simulink model "x5_Click"  (R2024b)
settings: Solver=VariableStepAuto  StartTime=0.0  StopTime=inf  RelTol=1e-3  EnableMultiTasking=on
libraries: simulink x6
(part 3 of 3)

== matlab function x5_Click/Robot_Direct_Kinematics1 ==
  data: q1 input; R06 output; q2 input; q3 input; q4 input; q5 input; q6 input; P6 output; J output
function [R06,P6,J] = Robot_Direct_Kinematics(q1,q2,q3,q4,q5,q6)
%#codegen

%    This function was generated by the Symbolic Math Toolbox version 24.2.
%    21-May-2025 19:19:44

% q1 = complex(q1);  % if required to enforce complex operations
% q2 = complex(q2);  % if required to enforce complex operations
% q3 = complex(q3);  % if required to enforce complex operations
% q4 = complex(q4);  % if required to enforce complex operations
% q5 = complex(q5);  % if required to enforce complex operations
% q6 = complex(q6);  % if required to enforce complex operations
et1 = cos(q5).*sin(q1).*sin(q3).*sqrt(sqrt(2.0)+2.0).*(-1.0./2.0)-(cos(q1).*cos(q2).*sin(q4).*sin(q6).*sqrt(-sqrt(2.0)+2.0))./2.0-(cos(q3).*cos(q4).*sin(q1).*sin(q6).*sqrt(-sqrt(2.0)+2.0))./2.0-(cos(q6).*sin(q1).*sin(q3).*sin(q5).*sqrt(-sqrt(2.0)+2.0))./2.0-(cos(q1).*cos(q3).*cos(q5).*sin(q2).*sqrt(sqrt(2.0)+2.0))./2.0-(cos(q1).*cos(q2).*cos(q4).*sin(q5).*sqrt(sqrt(2.0)+2.0))./2.0+(cos(q3).*sin(q1).*sin(q4).*sin(q5).*sqrt(sqrt(2.0)+2.0))./2.0;
et2 = (cos(q1).*cos(q2).*cos(q4).*cos(q5).*cos(q6).*sqrt(-sqrt(2.0)+2.0))./2.0-(cos(q1).*cos(q3).*cos(q6).*sin(q2).*sin(q5).*sqrt(-sqrt(2.0)+2.0))./2.0-(cos(q3).*cos(q5).*cos(q6).*sin(q1).*sin(q4).*sqrt(-sqrt(2.0)+2.0))./2.0+(cos(q1).*cos(q4).*sin(q2).*sin(q3).*sin(q6).*sqrt(-sqrt(2.0)+2.0))./2.0-(cos(q1).*sin(q2).*sin(q3).*sin(q4).*sin(q5).*sqrt(sqrt(2.0)+2.0))./2.0+(cos(q1).*cos(q5).*cos(q6).*sin(q2).*sin(q3).*sin(q4).*sqrt(-sqrt(2.0)+2.0))./2.0;
et3 = cos(q1).*cos(q5).*sin(q3).*sqrt(sqrt(2.0)+2.0).*(-1.0./2.0)-(cos(q1).*cos(q3).*cos(q4).*sin(q6).*sqrt(-sqrt(2.0)+2.0))./2.0-(cos(q1).*cos(q6).*sin(q3).*sin(q5).*sqrt(-sqrt(2.0)+2.0))./2.0+(cos(q2).*sin(q1).*sin(q4).*sin(q6).*sqrt(-sqrt(2.0)+2.0))./2.0+(cos(q3).*cos(q5).*sin(q1).*sin(q2).*sqrt(sqrt(2.0)+2.0))./2.0+(cos(q2).*cos(q4).*sin(q1).*sin(q5).*sqrt(sqrt(2.0)+2.0))./2.0+(cos(q1).*cos(q3).*sin(q4).*sin(q5).*sqrt(sqrt(2.0)+2.0))./2.0-(cos(q2).*cos(q4).*cos(q5).*cos(q6).*sin(q1).*sqrt(-sqrt(2.0)+2.0))./2.0;
et4 = cos(q1).*cos(q3).*cos(q5).*cos(q6).*sin(q4).*sqrt(-sqrt(2.0)+2.0).*(-1.0./2.0)+(cos(q3).*cos(q6).*sin(q1).*sin(q2).*sin(q5).*sqrt(-sqrt(2.0)+2.0))./2.0-(cos(q4).*sin(q1).*sin(q2).*sin(q3).*sin(q6).*sqrt(-sqrt(2.0)+2.0))./2.0+(sin(q1).*sin(q2).*sin(q3).*sin(q4).*sin(q5).*sqrt(sqrt(2.0)+2.0))./2.0-(cos(q5).*cos(q6).*sin(q1).*sin(q2).*sin(q3).*sin(q4).*sqrt(-sqrt(2.0)+2.0))./2.0;
et5 = cos(q5).*sin(q1).*sin(q3).*sqrt(-sqrt(2.0)+2.0).*(-1.0./2.0)-(cos(q1).*cos(q3).*cos(q5).*sin(q2).*sqrt(-sqrt(2.0)+2.0))./2.0-(cos(q1).*cos(q2).*cos(q4).*sin(q5).*sqrt(-sqrt(2.0)+2.0))./2.0+(cos(q3).*sin(q1).*sin(q4).*sin(q5).*sqrt(-sqrt(2.0)+2.0))./2.0+(cos(q1).*cos(q2).*sin(q4).*sin(q6).*sqrt(sqrt(2.0)+2.0))./2.0+(cos(q3).*cos(q4).*sin(q1).*sin(q6).*sqrt(sqrt(2.0)+2.0))./2.0+(cos(q6).*sin(q1).*sin(q3).*sin(q5).*sqrt(sqrt(2.0)+2.0))./2.0;
et6 = cos(q1).*sin(q2).*sin(q3).*sin(q4).*sin(q5).*sqrt(-sqrt(2.0)+2.0).*(-1.0./2.0)-(cos(q1).*cos(q2).*cos(q4).*cos(q5).*cos(q6).*sqrt(sqrt(2.0)+2.0))./2.0+(cos(q1).*cos(q3).*cos(q6).*sin(q2).*sin(q5).*sqrt(sqrt(2.0)+2.0))./2.0+(cos(q3).*cos(q5).*cos(q6).*sin(q1).*sin(q4).*sqrt(sqrt(2.0)+2.0))./2.0-(cos(q1).*cos(q4).*sin(q2).*sin(q3).*sin(q6).*sqrt(sqrt(2.0)+2.0))./2.0-(cos(q1).*cos(q5).*cos(q6).*sin(q2).*sin(q3).*sin(q4).*sqrt(sqrt(2.0)+2.0))./2.0;
et7 = cos(q1).*cos(q5).*sin(q3).*sqrt(-sqrt(2.0)+2.0).*(-1.0./2.0)+(cos(q3).*cos(q5).*sin(q1).*sin(q2).*sqrt(-sqrt(2.0)+2.0))./2.0+(cos(q2).*cos(q4).*sin(q1).*sin(q5).*sqrt(-sqrt(2.0)+2.0))./2.0+(cos(q1).*cos(q3).*sin(q4).*sin(q5).*sqrt(-sqrt(2.0)+2.0))./2.0+(cos(q1).*cos(q3).*cos(q4).*sin(q6).*sqrt(sqrt(2.0)+2.0))./2.0+(cos(q1).*cos(q6).*sin(q3).*sin(q5).*sqrt(sqrt(2.0)+2.0))./2.0-(cos(q2).*sin(q1).*sin(q4).*sin(q6).*sqrt(sqrt(2.0)+2.0))./2.0;
et8 = (sin(q1).*sin(q2).*sin(q3).*sin(q4).*sin(q5).*sqrt(-sqrt(2.0)+2.0))./2.0+(cos(q2).*cos(q4).*cos(q5).*cos(q6).*sin(q1).*sqrt(sqrt(2.0)+2.0))./2.0+(cos(q1).*cos(q3).*cos(q5).*cos(q6).*sin(q4).*sqrt(sqrt(2.0)+2.0))./2.0-(cos(q3).*cos(q6).*sin(q1).*sin(q2).*sin(q5).*sqrt(sqrt(2.0)+2.0))./2.0+(cos(q4).*sin(q1).*sin(q2).*sin(q3).*sin(q6).*sqrt(sqrt(2.0)+2.0))./2.0+(cos(q5).*cos(q6).*sin(q1).*sin(q2).*sin(q3).*sin(q4).*sqrt(sqrt(2.0)+2.0))./2.0;
mt1 = [cos(q1).*cos(q3).*cos(q4).*cos(q6)-cos(q2).*cos(q6).*sin(q1).*sin(q4)-cos(q1).*sin(q3).*sin(q5).*sin(q6)-cos(q2).*cos(q4).*cos(q5).*sin(q1).*sin(q6)-cos(q1).*cos(q3).*cos(q5).*sin(q4).*sin(q6)+cos(q4).*cos(q6).*sin(q1).*sin(q2).*sin(q3)+cos(q3).*sin(q1).*sin(q2).*sin(q5).*sin(q6)-cos(q5).*sin(q1).*sin(q2).*sin(q3).*sin(q4).*sin(q6),cos(q1).*cos(q2).*cos(q6).*sin(q4)+cos(q3).*cos(q4).*cos(q6).*sin(q1)-sin(q1).*sin(q3).*sin(q5).*sin(q6)+cos(q1).*cos(q2).*cos(q4).*cos(q5).*sin(q6)-cos(q1).*cos(q4).*cos(q6).*sin(q2).*sin(q3)-cos(q1).*cos(q3).*sin(q2).*sin(q5).*sin(q6)-cos(q3).*cos(q5).*sin(q1).*sin(q4).*sin(q6)+cos(q1).*cos(q5).*sin(q2).*sin(q3).*sin(q4).*sin(q6)];
mt2 = [cos(q6).*sin(q2).*sin(q4)+cos(q2).*cos(q4).*cos(q6).*sin(q3)+cos(q2).*cos(q3).*sin(q5).*sin(q6)+cos(q4).*cos(q5).*sin(q2).*sin(q6)-cos(q2).*cos(q5).*sin(q3).*sin(q4).*sin(q6),et3+et4,et1+et2];
mt3 = [cos(q4).*sin(q2).*sin(q5).*sqrt(sqrt(2.0)+2.0).*(-1.0./2.0)-(sin(q2).*sin(q4).*sin(q6).*sqrt(-sqrt(2.0)+2.0))./2.0+(cos(q2).*cos(q3).*cos(q5).*sqrt(sqrt(2.0)+2.0))./2.0+(cos(q2).*cos(q3).*cos(q6).*sin(q5).*sqrt(-sqrt(2.0)+2.0))./2.0+(cos(q4).*cos(q5).*cos(q6).*sin(q2).*sqrt(-sqrt(2.0)+2.0))./2.0-(cos(q2).*cos(q4).*sin(q3).*sin(q6).*sqrt(-sqrt(2.0)+2.0))./2.0+(cos(q2).*sin(q3).*sin(q4).*sin(q5).*sqrt(sqrt(2.0)+2.0))./2.0-(cos(q2).*cos(q5).*cos(q6).*sin(q3).*sin(q4).*sqrt(-sqrt(2.0)+2.0))./2.0];
mt4 = [et7+et8,et5+et6,(sin(q2).*sin(q4).*sin(q6).*sqrt(sqrt(2.0)+2.0))./2.0+(cos(q2).*cos(q3).*cos(q5).*sqrt(-sqrt(2.0)+2.0))./2.0-(cos(q4).*sin(q2).*sin(q5).*sqrt(-sqrt(2.0)+2.0))./2.0+(cos(q2).*sin(q3).*sin(q4).*sin(q5).*sqrt(-sqrt(2.0)+2.0))./2.0-(cos(q2).*cos(q3).*cos(q6).*sin(q5).*sqrt(sqrt(2.0)+2.0))./2.0-(cos(q4).*cos(q5).*cos(q6).*sin(q2).*sqrt(sqrt(2.0)+2.0))./2.0+(cos(q2).*cos(q4).*sin(q3).*sin(q6).*sqrt(sqrt(2.0)+2.0))./2.0+(cos(q2).*cos(q5).*cos(q6).*sin(q3).*sin(q4).*sqrt(sqrt(2.0)+2.0))./2.0];
R06 = reshape([mt1,mt2,mt3,mt4],3,3);
if nargout > 1
    et9 = sin(q2).*(-2.0./5.0)+(cos(q4).*sin(q2))./1.0e+1+(sin(q2).*sin(q4))./2.0+(cos(q2).*cos(q3).*cos(q5))./1.0e+1+(cos(q2).*cos(q4).*sin(q3))./2.0-(cos(q2).*sin(q3).*sin(q4))./1.0e+1-(cos(q4).*sin(q2).*sin(q5))./1.0e+1+sin(q2).*sin(q4).*sin(q6).*sqrt(sqrt(2.0)+2.0).*(3.0./4.0e+1)+cos(q2).*cos(q3).*cos(q5).*sqrt(-sqrt(2.0)+2.0).*(3.0./4.0e+1)-cos(q4).*sin(q2).*sin(q5).*sqrt(-sqrt(2.0)+2.0).*(3.0./4.0e+1)+(cos(q2).*sin(q3).*sin(q4).*sin(q5))./1.0e+1+cos(q2).*sin(q3).*sin(q4).*sin(q5).*sqrt(-sqrt(2.0)+2.0).*(3.0./4.0e+1);
    et10 = cos(q2).*cos(q3).*cos(q6).*sin(q5).*sqrt(sqrt(2.0)+2.0).*(-3.0./4.0e+1)-cos(q4).*cos(q5).*cos(q6).*sin(q2).*sqrt(sqrt(2.0)+2.0).*(3.0./4.0e+1)+cos(q2).*cos(q4).*sin(q3).*sin(q6).*sqrt(sqrt(2.0)+2.0).*(3.0./4.0e+1)+cos(q2).*cos(q5).*cos(q6).*sin(q3).*sin(q4).*sqrt(sqrt(2.0)+2.0).*(3.0./4.0e+1);
    et11 = cos(q1).*cos(q2).*(-2.0./5.0)+(cos(q1).*cos(q2).*cos(q4))./1.0e+1+(cos(q1).*cos(q2).*sin(q4))./2.0+(cos(q3).*cos(q4).*sin(q1))./2.0-(cos(q3).*sin(q1).*sin(q4))./1.0e+1-(cos(q5).*sin(q1).*sin(q3))./1.0e+1-cos(q5).*sin(q1).*sin(q3).*sqrt(-sqrt(2.0)+2.0).*(3.0./4.0e+1)-(cos(q1).*cos(q3).*cos(q5).*sin(q2))./1.0e+1-(cos(q1).*cos(q2).*cos(q4).*sin(q5))./1.0e+1-(cos(q1).*cos(q4).*sin(q2).*sin(q3))./2.0+(cos(q1).*sin(q2).*sin(q3).*sin(q4))./1.0e+1+(cos(q3).*sin(q1).*sin(q4).*sin(q5))./1.0e+1-cos(q1).*cos(q3).*cos(q5).*sin(q2).*sqrt(-sqrt(2.0)+2.0).*(3.0./4.0e+1);
    et12 = cos(q1).*cos(q2).*cos(q4).*sin(q5).*sqrt(-sqrt(2.0)+2.0).*(-3.0./4.0e+1)+cos(q3).*sin(q1).*sin(q4).*sin(q5).*sqrt(-sqrt(2.0)+2.0).*(3.0./4.0e+1)-(cos(q1).*sin(q2).*sin(q3).*sin(q4).*sin(q5))./1.0e+1+cos(q1).*cos(q2).*sin(q4).*sin(q6).*sqrt(sqrt(2.0)+2.0).*(3.0./4.0e+1)+cos(q3).*cos(q4).*sin(q1).*sin(q6).*sqrt(sqrt(2.0)+2.0).*(3.0./4.0e+1)+cos(q6).*sin(q1).*sin(q3).*sin(q5).*sqrt(sqrt(2.0)+2.0).*(3.0./4.0e+1)-cos(q1).*sin(q2).*sin(q3).*sin(q4).*sin(q5).*sqrt(-sqrt(2.0)+2.0).*(3.0./4.0e+1)-cos(q1).*cos(q2).*cos(q4).*cos(q5).*cos(q6).*sqrt(sqrt(2.0)+2.0).*(3.0./4.0e+1);
    et13 = cos(q1).*cos(q3).*cos(q6).*sin(q2).*sin(q5).*sqrt(sqrt(2.0)+2.0).*(3.0./4.0e+1)+cos(q3).*cos(q5).*cos(q6).*sin(q1).*sin(q4).*sqrt(sqrt(2.0)+2.0).*(3.0./4.0e+1)-cos(q1).*cos(q4).*sin(q2).*sin(q3).*sin(q6).*sqrt(sqrt(2.0)+2.0).*(3.0./4.0e+1)-cos(q1).*cos(q5).*cos(q6).*sin(q2).*sin(q3).*sin(q4).*sqrt(sqrt(2.0)+2.0).*(3.0./4.0e+1);
    et14 = cos(q2).*sin(q1).*(2.0./5.0)+(cos(q1).*cos(q3).*cos(q4))./2.0-(cos(q2).*cos(q4).*sin(q1))./1.0e+1-(cos(q1).*cos(q3).*sin(q4))./1.0e+1-(cos(q1).*cos(q5).*sin(q3))./1.0e+1-(cos(q2).*sin(q1).*sin(q4))./2.0-cos(q1).*cos(q5).*sin(q3).*sqrt(-sqrt(2.0)+2.0).*(3.0./4.0e+1)+(cos(q3).*cos(q5).*sin(q1).*sin(q2))./1.0e+1+(cos(q2).*cos(q4).*sin(q1).*sin(q5))./1.0e+1+(cos(q1).*cos(q3).*sin(q4).*sin(q5))./1.0e+1+(cos(q4).*sin(q1).*sin(q2).*sin(q3))./2.0-(sin(q1).*sin(q2).*sin(q3).*sin(q4))./1.0e+1+cos(q3).*cos(q5).*sin(q1).*sin(q2).*sqrt(-sqrt(2.0)+2.0).*(3.0./4.0e+1);
    et15 = cos(q2).*cos(q4).*sin(q1).*sin(q5).*sqrt(-sqrt(2.0)+2.0).*(3.0./4.0e+1)+cos(q1).*cos(q3).*sin(q4).*sin(q5).*sqrt(-sqrt(2.0)+2.0).*(3.0./4.0e+1)+(sin(q1).*sin(q2).*sin(q3).*sin(q4).*sin(q5))./1.0e+1+cos(q1).*cos(q3).*cos(q4).*sin(q6).*sqrt(sqrt(2.0)+2.0).*(3.0./4.0e+1)+cos(q1).*cos(q6).*sin(q3).*sin(q5).*sqrt(sqrt(2.0)+2.0).*(3.0./4.0e+1)-cos(q2).*sin(q1).*sin(q4).*sin(q6).*sqrt(sqrt(2.0)+2.0).*(3.0./4.0e+1)+sin(q1).*sin(q2).*sin(q3).*sin(q4).*sin(q5).*sqrt(-sqrt(2.0)+2.0).*(3.0./4.0e+1)+cos(q2).*cos(q4).*cos(q5).*cos(q6).*sin(q1).*sqrt(sqrt(2.0)+2.0).*(3.0./4.0e+1);
    et16 = cos(q1).*cos(q3).*cos(q5).*cos(q6).*sin(q4).*sqrt(sqrt(2.0)+2.0).*(3.0./4.0e+1)-cos(q3).*cos(q6).*sin(q1).*sin(q2).*sin(q5).*sqrt(sqrt(2.0)+2.0).*(3.0./4.0e+1)+cos(q4).*sin(q1).*sin(q2).*sin(q3).*sin(q6).*sqrt(sqrt(2.0)+2.0).*(3.0./4.0e+1)+cos(q5).*cos(q6).*sin(q1).*sin(q2).*sin(q3).*sin(q4).*sqrt(sqrt(2.0)+2.0).*(3.0./4.0e+1);
    P6 = [et14+et15+et16;et11+et12+et13;et9+et10];
end
if nargout > 2
    et17 = cos(q2).*sin(q1).*(2.0./5.0)+(cos(q1).*cos(q3).*cos(q4))./2.0-(cos(q2).*cos(q4).*sin(q1))./1.0e+1-(cos(q1).*cos(q3).*sin(q4))./1.0e+1-(cos(q1).*cos(q5).*sin(q3))./1.0e+1-(cos(q2).*sin(q1).*sin(q4))./2.0-cos(q1).*cos(q5).*sin(q3).*sqrt(-sqrt(2.0)+2.0).*(3.0./4.0e+1)+(cos(q3).*cos(q5).*sin(q1).*sin(q2))./1.0e+1+(cos(q2).*cos(q4).*sin(q1).*sin(q5))./1.0e+1+(cos(q1).*cos(q3).*sin(q4).*sin(q5))./1.0e+1+(cos(q4).*sin(q1).*sin(q2).*sin(q3))./2.0-(sin(q1).*sin(q2).*sin(q3).*sin(q4))./1.0e+1+cos(q3).*cos(q5).*sin(q1).*sin(q2).*sqrt(-sqrt(2.0)+2.0).*(3.0./4.0e+1);
    et18 = cos(q2).*cos(q4).*sin(q1).*sin(q5).*sqrt(-sqrt(2.0)+2.0).*(3.0./4.0e+1)+cos(q1).*cos(q3).*sin(q4).*sin(q5).*sqrt(-sqrt(2.0)+2.0).*(3.0./4.0e+1)+(sin(q1).*sin(q2).*sin(q3).*sin(q4).*sin(q5))./1.0e+1+cos(q1).*cos(q3).*cos(q4).*sin(q6).*sqrt(sqrt(2.0)+2.0).*(3.0./4.0e+1)+cos(q1).*cos(q6).*sin(q3).*sin(q5).*sqrt(sqrt(2.0)+2.0).*(3.0./4.0e+1)-cos(q2).*sin(q1).*sin(q4).*sin(q6).*sqrt(sqrt(2.0)+2.0).*(3.0./4.0e+1)+sin(q1).*sin(q2).*sin(q3).*sin(q4).*sin(q5).*sqrt(-sqrt(2.0)+2.0).*(3.0./4.0e+1)+cos(q2).*cos(q4).*cos(q5).*cos(q6).*sin(q1).*sqrt(sqrt(2.0)+2.0).*(3.0./4.0e+1);
    et19 = cos(q1).*cos(q3).*cos(q5).*cos(q6).*sin(q4).*sqrt(sqrt(2.0)+2.0).*(3.0./4.0e+1)-cos(q3).*cos(q6).*sin(q1).*sin(q2).*sin(q5).*sqrt(sqrt(2.0)+2.0).*(3.0./4.0e+1)+cos(q4).*sin(q1).*sin(q2).*sin(q3).*sin(q6).*sqrt(sqrt(2.0)+2.0).*(3.0./4.0e+1)+cos(q5).*cos(q6).*sin(q1).*sin(q2).*sin(q3).*sin(q4).*sqrt(sqrt(2.0)+2.0).*(3.0./4.0e+1);
    et20 = cos(q1).*cos(q2).*(2.0./5.0)-(cos(q1).*cos(q2).*cos(q4))./1.0e+1-(cos(q1).*cos(q2).*sin(q4))./2.0-(cos(q3).*cos(q4).*sin(q1))./2.0+(cos(q3).*sin(q1).*sin(q4))./1.0e+1+(cos(q5).*sin(q1).*sin(q3))./1.0e+1+cos(q5).*sin(q1).*sin(q3).*sqrt(-sqrt(2.0)+2.0).*(3.0./4.0e+1)+(cos(q1).*cos(q3).*cos(q5).*sin(q2))./1.0e+1+(cos(q1).*cos(q2).*cos(q4).*sin(q5))./1.0e+1+(cos(q1).*cos(q4).*sin(q2).*sin(q3))./2.0-(cos(q1).*sin(q2).*sin(q3).*sin(q4))./1.0e+1-(cos(q3).*sin(q1).*sin(q4).*sin(q5))./1.0e+1+cos(q1).*cos(q3).*cos(q5).*sin(q2).*sqrt(-sqrt(2.0)+2.0).*(3.0./4.0e+1);
    et21 = cos(q1).*cos(q2).*cos(q4).*sin(q5).*sqrt(-sqrt(2.0)+2.0).*(3.0./4.0e+1)-cos(q3).*sin(q1).*sin(q4).*sin(q5).*sqrt(-sqrt(2.0)+2.0).*(3.0./4.0e+1)+(cos(q1).*sin(q2).*sin(q3).*sin(q4).*sin(q5))./1.0e+1-cos(q1).*cos(q2).*sin(q4).*sin(q6).*sqrt(sqrt(2.0)+2.0).*(3.0./4.0e+1)-cos(q3).*cos(q4).*sin(q1).*sin(q6).*sqrt(sqrt(2.0)+2.0).*(3.0./4.0e+1)-cos(q6).*sin(q1).*sin(q3).*sin(q5).*sqrt(sqrt(2.0)+2.0).*(3.0./4.0e+1)+cos(q1).*sin(q2).*sin(q3).*sin(q4).*sin(q5).*sqrt(-sqrt(2.0)+2.0).*(3.0./4.0e+1)+cos(q1).*cos(q2).*cos(q4).*cos(q5).*cos(q6).*sqrt(sqrt(2.0)+2.0).*(3.0./4.0e+1);
    et22 = cos(q1).*cos(q3).*cos(q6).*sin(q2).*sin(q5).*sqrt(sqrt(2.0)+2.0).*(-3.0./4.0e+1)-cos(q3).*cos(q5).*cos(q6).*sin(q1).*sin(q4).*sqrt(sqrt(2.0)+2.0).*(3.0./4.0e+1)+cos(q1).*cos(q4).*sin(q2).*sin(q3).*sin(q6).*sqrt(sqrt(2.0)+2.0).*(3.0./4.0e+1)+cos(q1).*cos(q5).*cos(q6).*sin(q2).*sin(q3).*sin(q4).*sqrt(sqrt(2.0)+2.0).*(3.0./4.0e+1);
    et23 = cos(q2).*(-2.0./5.0)+(cos(q2).*cos(q4))./1.0e+1+(cos(q2).*sin(q4))./2.0+(sin(q2).*sin(q3).*sin(q4))./1.0e+1-(cos(q3).*cos(q5).*sin(q2))./1.0e+1-(cos(q2).*cos(q4).*sin(q5))./1.0e+1-(cos(q4).*sin(q2).*sin(q3))./2.0+cos(q2).*sin(q4).*sin(q6).*sqrt(sqrt(2.0)+2.0).*(3.0./4.0e+1)-cos(q3).*cos(q5).*sin(q2).*sqrt(-sqrt(2.0)+2.0).*(3.0./4.0e+1)-cos(q2).*cos(q4).*sin(q5).*sqrt(-sqrt(2.0)+2.0).*(3.0./4.0e+1)-(sin(q2).*sin(q3).*sin(q4).*sin(q5))./1.0e+1-sin(q2).*sin(q3).*sin(q4).*sin(q5).*sqrt(-sqrt(2.0)+2.0).*(3.0./4.0e+1);
    et24 = cos(q2).*cos(q4).*cos(q5).*cos(q6).*sqrt(sqrt(2.0)+2.0).*(-3.0./4.0e+1)+cos(q3).*cos(q6).*sin(q2).*sin(q5).*sqrt(sqrt(2.0)+2.0).*(3.0./4.0e+1)-cos(q4).*sin(q2).*sin(q3).*sin(q6).*sqrt(sqrt(2.0)+2.0).*(3.0./4.0e+1)-cos(q5).*cos(q6).*sin(q2).*sin(q3).*sin(q4).*sqrt(sqrt(2.0)+2.0).*(3.0./4.0e+1);
    et25 = sin(q2).*-1.6e+1+cos(q4).*sin(q2).*4.0+sin(q2).*sin(q4).*2.0e+1+cos(q2).*cos(q3).*cos(q5).*4.0+cos(q2).*cos(q4).*sin(q3).*2.0e+1-cos(q2).*sin(q3).*sin(q4).*4.0-cos(q4).*sin(q2).*sin(q5).*4.0+sin(q2).*sin(q4).*sin(q6).*sqrt(sqrt(2.0)+2.0).*3.0+cos(q2).*cos(q3).*cos(q5).*sqrt(-sqrt(2.0)+2.0).*3.0-cos(q4).*sin(q2).*sin(q5).*sqrt(-sqrt(2.0)+2.0).*3.0+cos(q2).*sin(q3).*sin(q4).*sin(q5).*4.0+cos(q2).*sin(q3).*sin(q4).*sin(q5).*sqrt(-sqrt(2.0)+2.0).*3.0-cos(q2).*cos(q3).*cos(q6).*sin(q5).*sqrt(sqrt(2.0)+2.0).*3.0-cos(q4).*cos(q5).*cos(q6).*sin(q2).*sqrt(sqrt(2.0)+2.0).*3.0;
    et26 = cos(q2).*cos(q4).*sin(q3).*sin(q6).*sqrt(sqrt(2.0)+2.0).*3.0+cos(q2).*cos(q5).*cos(q6).*sin(q3).*sin(q4).*sqrt(sqrt(2.0)+2.0).*3.0;
    et27 = sin(q2).*-1.6e+1+cos(q4).*sin(q2).*4.0+sin(q2).*sin(q4).*2.0e+1+cos(q2).*cos(q3).*cos(q5).*4.0+cos(q2).*cos(q4).*sin(q3).*2.0e+1-cos(q2).*sin(q3).*sin(q4).*4.0-cos(q4).*sin(q2).*sin(q5).*4.0+sin(q2).*sin(q4).*sin(q6).*sqrt(sqrt(2.0)+2.0).*3.0+cos(q2).*cos(q3).*cos(q5).*sqrt(-sqrt(2.0)+2.0).*3.0-cos(q4).*sin(q2).*sin(q5).*sqrt(-sqrt(2.0)+2.0).*3.0+cos(q2).*sin(q3).*sin(q4).*sin(q5).*4.0+cos(q2).*sin(q3).*sin(q4).*sin(q5).*sqrt(-sqrt(2.0)+2.0).*3.0-cos(q2).*cos(q3).*cos(q6).*sin(q5).*sqrt(sqrt(2.0)+2.0).*3.0-cos(q4).*cos(q5).*cos(q6).*sin(q2).*sqrt(sqrt(2.0)+2.0).*3.0;
    et28 = cos(q2).*cos(q4).*sin(q3).*sin(q6).*sqrt(sqrt(2.0)+2.0).*3.0+cos(q2).*cos(q5).*cos(q6).*sin(q3).*sin(q4).*sqrt(sqrt(2.0)+2.0).*3.0;
    et29 = (sin(q1).*sin(q3).*sin(q4))./1.0e+1-(cos(q3).*cos(q5).*sin(q1))./1.0e+1-(cos(q4).*sin(q1).*sin(q3))./2.0-cos(q3).*cos(q5).*sin(q1).*sqrt(-sqrt(2.0)+2.0).*(3.0./4.0e+1)-(cos(q1).*cos(q3).*cos(q4).*sin(q2))./2.0+(cos(q1).*cos(q3).*sin(q2).*sin(q4))./1.0e+1+(cos(q1).*cos(q5).*sin(q2).*sin(q3))./1.0e+1-(sin(q1).*sin(q3).*sin(q4).*sin(q5))./1.0e+1+cos(q1).*cos(q5).*sin(q2).*sin(q3).*sqrt(-sqrt(2.0)+2.0).*(3.0./4.0e+1)-sin(q1).*sin(q3).*sin(q4).*sin(q5).*sqrt(-sqrt(2.0)+2.0).*(3.0./4.0e+1)-(cos(q1).*cos(q3).*sin(q2).*sin(q4).*sin(q5))./1.0e+1;
    et30 = cos(q3).*cos(q6).*sin(q1).*sin(q5).*sqrt(sqrt(2.0)+2.0).*(3.0./4.0e+1)-cos(q4).*sin(q1).*sin(q3).*sin(q6).*sqrt(sqrt(2.0)+2.0).*(3.0./4.0e+1)-cos(q1).*cos(q3).*sin(q2).*sin(q4).*sin(q5).*sqrt(-sqrt(2.0)+2.0).*(3.0./4.0e+1)-cos(q1).*cos(q3).*cos(q4).*sin(q2).*sin(q6).*sqrt(sqrt(2.0)+2.0).*(3.0./4.0e+1)-cos(q1).*cos(q6).*sin(q2).*sin(q3).*sin(q5).*sqrt(sqrt(2.0)+2.0).*(3.0./4.0e+1)-cos(q5).*cos(q6).*sin(q1).*sin(q3).*sin(q4).*sqrt(sqrt(2.0)+2.0).*(3.0./4.0e+1)-cos(q1).*cos(q3).*cos(q5).*cos(q6).*sin(q2).*sin(q4).*sqrt(sqrt(2.0)+2.0).*(3.0./4.0e+1);
    et31 = cos(q1).*cos(q3).*cos(q5).*(-1.0./1.0e+1)-(cos(q1).*cos(q4).*sin(q3))./2.0+(cos(q1).*sin(q3).*sin(q4))./1.0e+1-cos(q1).*cos(q3).*cos(q5).*sqrt(-sqrt(2.0)+2.0).*(3.0./4.0e+1)+(cos(q3).*cos(q4).*sin(q1).*sin(q2))./2.0-(cos(q3).*sin(q1).*sin(q2).*sin(q4))./1.0e+1-(cos(q5).*sin(q1).*sin(q2).*sin(q3))./1.0e+1-(cos(q1).*sin(q3).*sin(q4).*sin(q5))./1.0e+1-cos(q5).*sin(q1).*sin(q2).*sin(q3).*sqrt(-sqrt(2.0)+2.0).*(3.0./4.0e+1)-cos(q1).*sin(q3).*sin(q4).*sin(q5).*sqrt(-sqrt(2.0)+2.0).*(3.0./4.0e+1)+(cos(q3).*sin(q1).*sin(q2).*sin(q4).*sin(q5))./1.0e+1;
    et32 = cos(q1).*cos(q3).*cos(q6).*sin(q5).*sqrt(sqrt(2.0)+2.0).*(3.0./4.0e+1)-cos(q1).*cos(q4).*sin(q3).*sin(q6).*sqrt(sqrt(2.0)+2.0).*(3.0./4.0e+1)+cos(q3).*sin(q1).*sin(q2).*sin(q4).*sin(q5).*sqrt(-sqrt(2.0)+2.0).*(3.0./4.0e+1)-cos(q1).*cos(q5).*cos(q6).*sin(q3).*sin(q4).*sqrt(sqrt(2.0)+2.0).*(3.0./4.0e+1)+cos(q3).*cos(q4).*sin(q1).*sin(q2).*sin(q6).*sqrt(sqrt(2.0)+2.0).*(3.0./4.0e+1)+cos(q6).*sin(q1).*sin(q2).*sin(q3).*sin(q5).*sqrt(sqrt(2.0)+2.0).*(3.0./4.0e+1)+cos(q3).*cos(q5).*cos(q6).*sin(q1).*sin(q2).*sin(q4).*sqrt(sqrt(2.0)+2.0).*(3.0./4.0e+1);
    et33 = (cos(q4).*sin(q2))./2.0-(sin(q2).*sin(q4))./1.0e+1+(sin(q2).*sin(q4).*sin(q5))./1.0e+1-(cos(q2).*cos(q4).*sin(q3))./1.0e+1-(cos(q2).*sin(q3).*sin(q4))./2.0+cos(q4).*sin(q2).*sin(q6).*sqrt(sqrt(2.0)+2.0).*(3.0./4.0e+1)+sin(q2).*sin(q4).*sin(q5).*sqrt(-sqrt(2.0)+2.0).*(3.0./4.0e+1)+(cos(q2).*cos(q4).*sin(q3).*sin(q5))./1.0e+1+cos(q2).*cos(q4).*sin(q3).*sin(q5).*sqrt(-sqrt(2.0)+2.0).*(3.0./4.0e+1)+cos(q5).*cos(q6).*sin(q2).*sin(q4).*sqrt(sqrt(2.0)+2.0).*(3.0./4.0e+1)-cos(q2).*sin(q3).*sin(q4).*sin(q6).*sqrt(sqrt(2.0)+2.0).*(3.0./4.0e+1);
    et34 = cos(q2).*cos(q4).*cos(q5).*cos(q6).*sin(q3).*sqrt(sqrt(2.0)+2.0).*(3.0./4.0e+1);
    et35 = (cos(q1).*cos(q2).*cos(q4))./2.0-(cos(q1).*cos(q2).*sin(q4))./1.0e+1-(cos(q3).*cos(q4).*sin(q1))./1.0e+1-(cos(q3).*sin(q1).*sin(q4))./2.0+(cos(q1).*cos(q4).*sin(q2).*sin(q3))./1.0e+1+(cos(q1).*cos(q2).*sin(q4).*sin(q5))./1.0e+1+(cos(q3).*cos(q4).*sin(q1).*sin(q5))./1.0e+1+(cos(q1).*sin(q2).*sin(q3).*sin(q4))./2.0+cos(q1).*cos(q2).*sin(q4).*sin(q5).*sqrt(-sqrt(2.0)+2.0).*(3.0./4.0e+1)+cos(q3).*cos(q4).*sin(q1).*sin(q5).*sqrt(-sqrt(2.0)+2.0).*(3.0./4.0e+1)-(cos(q1).*cos(q4).*sin(q2).*sin(q3).*sin(q5))./1.0e+1+cos(q1).*cos(q2).*cos(q4).*sin(q6).*sqrt(sqrt(2.0)+2.0).*(3.0./4.0e+1);
    et36 = cos(q3).*sin(q1).*sin(q4).*sin(q6).*sqrt(sqrt(2.0)+2.0).*(-3.0./4.0e+1)-cos(q1).*cos(q4).*sin(q2).*sin(q3).*sin(q5).*sqrt(-sqrt(2.0)+2.0).*(3.0./4.0e+1)+cos(q1).*cos(q2).*cos(q5).*cos(q6).*sin(q4).*sqrt(sqrt(2.0)+2.0).*(3.0./4.0e+1)+cos(q3).*cos(q4).*cos(q5).*cos(q6).*sin(q1).*sqrt(sqrt(2.0)+2.0).*(3.0./4.0e+1)+cos(q1).*sin(q2).*sin(q3).*sin(q4).*sin(q6).*sqrt(sqrt(2.0)+2.0).*(3.0./4.0e+1)-cos(q1).*cos(q4).*cos(q5).*cos(q6).*sin(q2).*sin(q3).*sqrt(sqrt(2.0)+2.0).*(3.0./4.0e+1);
    et37 = cos(q1).*cos(q3).*cos(q4).*(-1.0./1.0e+1)-(cos(q2).*cos(q4).*sin(q1))./2.0-(cos(q1).*cos(q3).*sin(q4))./2.0+(cos(q2).*sin(q1).*sin(q4))./1.0e+1+(cos(q1).*cos(q3).*cos(q4).*sin(q5))./1.0e+1-(cos(q4).*sin(q1).*sin(q2).*sin(q3))./1.0e+1-(cos(q2).*sin(q1).*sin(q4).*sin(q5))./1.0e+1-(sin(q1).*sin(q2).*sin(q3).*sin(q4))./2.0+cos(q1).*cos(q3).*cos(q4).*sin(q5).*sqrt(-sqrt(2.0)+2.0).*(3.0./4.0e+1)-cos(q2).*sin(q1).*sin(q4).*sin(q5).*sqrt(-sqrt(2.0)+2.0).*(3.0./4.0e+1)+(cos(q4).*sin(q1).*sin(q2).*sin(q3).*sin(q5))./1.0e+1-cos(q2).*cos(q4).*sin(q1).*sin(q6).*sqrt(sqrt(2.0)+2.0).*(3.0./4.0e+1);
    et38 = cos(q1).*cos(q3).*sin(q4).*sin(q6).*sqrt(sqrt(2.0)+2.0).*(-3.0./4.0e+1)+cos(q4).*sin(q1).*sin(q2).*sin(q3).*sin(q5).*sqrt(-sqrt(2.0)+2.0).*(3.0./4.0e+1)+cos(q1).*cos(q3).*cos(q4).*cos(q5).*cos(q6).*sqrt(sqrt(2.0)+2.0).*(3.0./4.0e+1)-cos(q2).*cos(q5).*cos(q6).*sin(q1).*sin(q4).*sqrt(sqrt(2.0)+2.0).*(3.0./4.0e+1)-sin(q1).*sin(q2).*sin(q3).*sin(q4).*sin(q6).*sqrt(sqrt(2.0)+2.0).*(3.0./4.0e+1)+cos(q4).*cos(q5).*cos(q6).*sin(q1).*sin(q2).*sin(q3).*sqrt(sqrt(2.0)+2.0).*(3.0./4.0e+1);
    et39 = (sin(q1).*sin(q3).*sin(q5))./1.0e+1+sin(q1).*sin(q3).*sin(q5).*sqrt(-sqrt(2.0)+2.0).*(3.0./4.0e+1)-(cos(q1).*cos(q2).*cos(q4).*cos(q5))./1.0e+1+(cos(q1).*cos(q3).*sin(q2).*sin(q5))./1.0e+1+(cos(q3).*cos(q5).*sin(q1).*sin(q4))./1.0e+1-cos(q1).*cos(q2).*cos(q4).*cos(q5).*sqrt(-sqrt(2.0)+2.0).*(3.0./4.0e+1)+cos(q1).*cos(q3).*sin(q2).*sin(q5).*sqrt(-sqrt(2.0)+2.0).*(3.0./4.0e+1)+cos(q3).*cos(q5).*sin(q1).*sin(q4).*sqrt(-sqrt(2.0)+2.0).*(3.0./4.0e+1)-(cos(q1).*cos(q5).*sin(q2).*sin(q3).*sin(q4))./1.0e+1+cos(q5).*cos(q6).*sin(q1).*sin(q3).*sqrt(sqrt(2.0)+2.0).*(3.0./4.0e+1);
    et40 = cos(q1).*cos(q5).*sin(q2).*sin(q3).*sin(q4).*sqrt(-sqrt(2.0)+2.0).*(-3.0./4.0e+1)+cos(q1).*cos(q3).*cos(q5).*cos(q6).*sin(q2).*sqrt(sqrt(2.0)+2.0).*(3.0./4.0e+1)+cos(q1).*cos(q2).*cos(q4).*cos(q6).*sin(q5).*sqrt(sqrt(2.0)+2.0).*(3.0./4.0e+1)-cos(q3).*cos(q6).*sin(q1).*sin(q4).*sin(q5).*sqrt(sqrt(2.0)+2.0).*(3.0./4.0e+1)+cos(q1).*cos(q6).*sin(q2).*sin(q3).*sin(q4).*sin(q5).*sqrt(sqrt(2.0)+2.0).*(3.0./4.0e+1);
    et41 = (cos(q1).*sin(q3).*sin(q5))./1.0e+1+cos(q1).*sin(q3).*sin(q5).*sqrt(-sqrt(2.0)+2.0).*(3.0./4.0e+1)+(cos(q2).*cos(q4).*cos(q5).*sin(q1))./1.0e+1+(cos(q1).*cos(q3).*cos(q5).*sin(q4))./1.0e+1-(cos(q3).*sin(q1).*sin(q2).*sin(q5))./1.0e+1+cos(q2).*cos(q4).*cos(q5).*sin(q1).*sqrt(-sqrt(2.0)+2.0).*(3.0./4.0e+1)+cos(q1).*cos(q3).*cos(q5).*sin(q4).*sqrt(-sqrt(2.0)+2.0).*(3.0./4.0e+1)-cos(q3).*sin(q1).*sin(q2).*sin(q5).*sqrt(-sqrt(2.0)+2.0).*(3.0./4.0e+1)+(cos(q5).*sin(q1).*sin(q2).*sin(q3).*sin(q4))./1.0e+1+cos(q1).*cos(q5).*cos(q6).*sin(q3).*sqrt(sqrt(2.0)+2.0).*(3.0./4.0e+1);
    et42 = cos(q5).*sin(q1).*sin(q2).*sin(q3).*sin(q4).*sqrt(-sqrt(2.0)+2.0).*(3.0./4.0e+1)-cos(q3).*cos(q5).*cos(q6).*sin(q1).*sin(q2).*sqrt(sqrt(2.0)+2.0).*(3.0./4.0e+1)-cos(q2).*cos(q4).*cos(q6).*sin(q1).*sin(q5).*sqrt(sqrt(2.0)+2.0).*(3.0./4.0e+1)-cos(q1).*cos(q3).*cos(q6).*sin(q4).*sin(q5).*sqrt(sqrt(2.0)+2.0).*(3.0./4.0e+1)-cos(q6).*sin(q1).*sin(q2).*sin(q3).*sin(q4).*sin(q5).*sqrt(sqrt(2.0)+2.0).*(3.0./4.0e+1);
    et43 = sin(q1).*sin(q3).*sin(q5).*sin(q6).*sqrt(sqrt(2.0)+2.0).*(-3.0./4.0e+1)+cos(q1).*cos(q2).*cos(q6).*sin(q4).*sqrt(sqrt(2.0)+2.0).*(3.0./4.0e+1)+cos(q3).*cos(q4).*cos(q6).*sin(q1).*sqrt(sqrt(2.0)+2.0).*(3.0./4.0e+1)+cos(q1).*cos(q2).*cos(q4).*cos(q5).*sin(q6).*sqrt(sqrt(2.0)+2.0).*(3.0./4.0e+1)-cos(q1).*cos(q4).*cos(q6).*sin(q2).*sin(q3).*sqrt(sqrt(2.0)+2.0).*(3.0./4.0e+1)-cos(q1).*cos(q3).*sin(q2).*sin(q5).*sin(q6).*sqrt(sqrt(2.0)+2.0).*(3.0./4.0e+1)-cos(q3).*cos(q5).*sin(q1).*sin(q4).*sin(q6).*sqrt(sqrt(2.0)+2.0).*(3.0./4.0e+1);
    et44 = cos(q1).*cos(q5).*sin(q2).*sin(q3).*sin(q4).*sin(q6).*sqrt(sqrt(2.0)+2.0).*(3.0./4.0e+1);
    et45 = cos(q1).*cos(q3).*cos(q4).*cos(q6).*sqrt(sqrt(2.0)+2.0).*(3.0./4.0e+1)-cos(q2).*cos(q6).*sin(q1).*sin(q4).*sqrt(sqrt(2.0)+2.0).*(3.0./4.0e+1)-cos(q1).*sin(q3).*sin(q5).*sin(q6).*sqrt(sqrt(2.0)+2.0).*(3.0./4.0e+1)-cos(q2).*cos(q4).*cos(q5).*sin(q1).*sin(q6).*sqrt(sqrt(2.0)+2.0).*(3.0./4.0e+1)-cos(q1).*cos(q3).*cos(q5).*sin(q4).*sin(q6).*sqrt(sqrt(2.0)+2.0).*(3.0./4.0e+1)+cos(q4).*cos(q6).*sin(q1).*sin(q2).*sin(q3).*sqrt(sqrt(2.0)+2.0).*(3.0./4.0e+1)+cos(q3).*sin(q1).*sin(q2).*sin(q5).*sin(q6).*sqrt(sqrt(2.0)+2.0).*(3.0./4.0e+1);
    et46 = cos(q5).*sin(q1).*sin(q2).*sin(q3).*sin(q4).*sin(q6).*sqrt(sqrt(2.0)+2.0).*(-3.0./4.0e+1);
    mt5 = [et20+et21+et22,et17+et18+et19,0.0,0.0,0.0,1.0,(sin(q1).*(et27+et28))./4.0e+1,cos(q1).*(et25+et26).*(-1.0./4.0e+1),et23+et24,cos(q1),sin(q1),0.0,et31+et32,et29+et30,(cos(q2).*(cos(q3).*cos(q4).*2.0e+1-cos(q3).*sin(q4).*4.0-cos(q5).*sin(q3).*4.0-cos(q5).*sin(q3).*sqrt(-sqrt(2.0)+2.0).*3.0+cos(q3).*sin(q4).*sin(q5).*4.0+cos(q3).*cos(q4).*sin(q6).*sqrt(sqrt(2.0)+2.0).*3.0+cos(q6).*sin(q3).*sin(q5).*sqrt(sqrt(2.0)+2.0).*3.0+cos(q3).*sin(q4).*sin(q5).*sqrt(-sqrt(2.0)+2.0).*3.0+cos(q3).*cos(q5).*cos(q6).*sin(q4).*sqrt(sqrt(2.0)+2.0).*3.0))./4.0e+1,cos(q2).*sin(q1),-cos(q1).*cos(q2)];
    mt6 = [-sin(q2),et37+et38,et35+et36,et33+et34,-cos(q1).*sin(q3)+cos(q3).*sin(q1).*sin(q2),-sin(q1).*sin(q3)-cos(q1).*cos(q3).*sin(q2),cos(q2).*cos(q3),et41+et42,et39+et40];
    mt7 = [cos(q2).*cos(q3).*sin(q5).*(-1.0./1.0e+1)-(cos(q4).*cos(q5).*sin(q2))./1.0e+1-cos(q2).*cos(q3).*sin(q5).*sqrt(-sqrt(2.0)+2.0).*(3.0./4.0e+1)-cos(q4).*cos(q5).*sin(q2).*sqrt(-sqrt(2.0)+2.0).*(3.0./4.0e+1)+(cos(q2).*cos(q5).*sin(q3).*sin(q4))./1.0e+1+cos(q2).*cos(q5).*sin(q3).*sin(q4).*sqrt(-sqrt(2.0)+2.0).*(3.0./4.0e+1)-cos(q2).*cos(q3).*cos(q5).*cos(q6).*sqrt(sqrt(2.0)+2.0).*(3.0./4.0e+1)+cos(q4).*cos(q6).*sin(q2).*sin(q5).*sqrt(sqrt(2.0)+2.0).*(3.0./4.0e+1)-cos(q2).*cos(q6).*sin(q3).*sin(q4).*sin(q5).*sqrt(sqrt(2.0)+2.0).*(3.0./4.0e+1)];
    mt8 = [cos(q1).*cos(q3).*cos(q4)-cos(q2).*sin(q1).*sin(q4)+cos(q4).*sin(q1).*sin(q2).*sin(q3),cos(q1).*cos(q2).*sin(q4)+cos(q3).*cos(q4).*sin(q1)-cos(q1).*cos(q4).*sin(q2).*sin(q3),sin(q2).*sin(q4)+cos(q2).*cos(q4).*sin(q3),et45+et46,et43+et44,cos(q6).*sin(q2).*sin(q4).*sqrt(sqrt(2.0)+2.0).*(3.0./4.0e+1)+cos(q2).*cos(q4).*cos(q6).*sin(q3).*sqrt(sqrt(2.0)+2.0).*(3.0./4.0e+1)+cos(q2).*cos(q3).*sin(q5).*sin(q6).*sqrt(sqrt(2.0)+2.0).*(3.0./4.0e+1)+cos(q4).*cos(q5).*sin(q2).*sin(q6).*sqrt(sqrt(2.0)+2.0).*(3.0./4.0e+1)-cos(q2).*cos(q5).*sin(q3).*sin(q4).*sin(q6).*sqrt(sqrt(2.0)+2.0).*(3.0./4.0e+1)];
    mt9 = [-cos(q1).*cos(q5).*sin(q3)+cos(q3).*cos(q5).*sin(q1).*sin(q2)+cos(q2).*cos(q4).*sin(q1).*sin(q5)+cos(q1).*cos(q3).*sin(q4).*sin(q5)+sin(q1).*sin(q2).*sin(q3).*sin(q4).*sin(q5),-cos(q5).*sin(q1).*sin(q3)-cos(q1).*cos(q3).*cos(q5).*sin(q2)-cos(q1).*cos(q2).*cos(q4).*sin(q5)+cos(q3).*sin(q1).*sin(q4).*sin(q5)-cos(q1).*sin(q2).*sin(q3).*sin(q4).*sin(q5),cos(q2).*cos(q3).*cos(q5)-cos(q4).*sin(q2).*sin(q5)+cos(q2).*sin(q3).*sin(q4).*sin(q5)];
    J = reshape([mt5,mt6,mt7,mt8,mt9],6,6);
end
end
